simulink model "sin_critical"  (R2019a)
settings: Solver=VariableStepAuto  StartTime=0.0  StopTime=10.0  RelTol=1e-3
libraries: dsparch4 x2
settings Model: Creator=LeoLi  LastModifiedBy=LeoLi

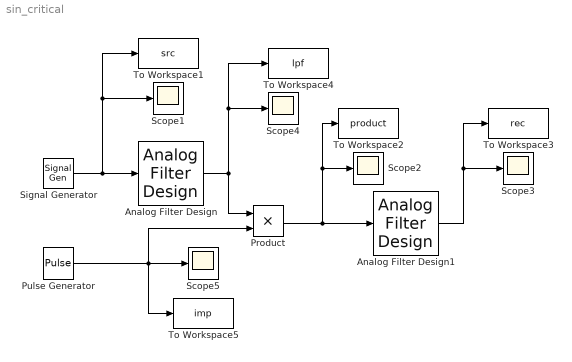
== system sin_critical ==
  Analog Filter Design : dsparch4/Analog Filter Design  method=Butterworth  filttype=Lowpass  N=8  Wlo=30  Whi=80  Rp=2  Rs=40
  Analog Filter Design1 : dsparch4/Analog Filter Design  method=Butterworth  filttype=Lowpass  N=8  Wlo=4*pi  Whi=80  Rp=2  Rs=40
  Product : Product
  Pulse Generator : DiscretePulseGenerator  PulseType=Time based  Amplitude=40*sqrt(2)  Period=0.5
  Scope{1..5} (5 alike) : Scope
  Signal Generator : SignalGenerator
  To Workspace1 : ToWorkspace  VariableName=src  SampleTime=-1
      settings: Save2DSignal=2-D array (concatenate along first dimension)
  To Workspace2 : ToWorkspace  VariableName=product  SampleTime=-1
      settings: Save2DSignal=2-D array (concatenate along first dimension)
  To Workspace3 : ToWorkspace  VariableName=rec  SampleTime=-1
      settings: Save2DSignal=2-D array (concatenate along first dimension)
  To Workspace4 : ToWorkspace  VariableName=lpf  SampleTime=-1
      settings: Save2DSignal=2-D array (concatenate along first dimension)
  To Workspace5 : ToWorkspace  VariableName=imp  SampleTime=-1
      settings: Save2DSignal=2-D array (concatenate along first dimension)
  wires:
  Signal Generator/1 -> Scope1/1, To Workspace1/1, Analog Filter Design/1
  Pulse Generator/1 -> To Workspace5/1, Scope5/1, Product/2
  Product/1 -> Scope2/1, To Workspace2/1, Analog Filter Design1/1
  Analog Filter Design1/1 -> Scope3/1, To Workspace3/1
  Analog Filter Design/1 -> Scope4/1, To Workspace4/1, Product/1
